simulink model "SH_control_harness1"  (R2023b)
settings: Solver=VariableStepAuto  StartTime=0.0  StopTime=inf  RelTol=1e-3
settings Model: Creator=Veimar  LastModifiedBy=Veimar

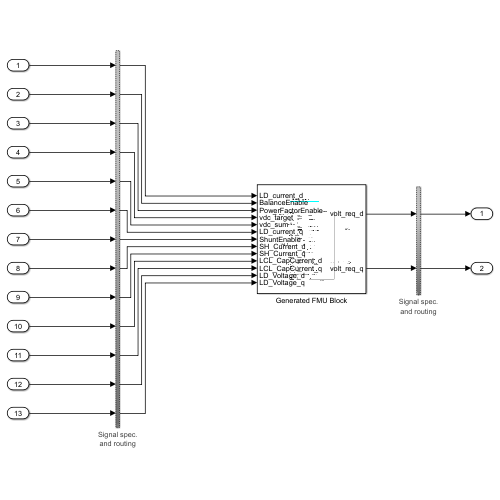
[thumbnail: Simulink's stored preview of the top-level diagram]
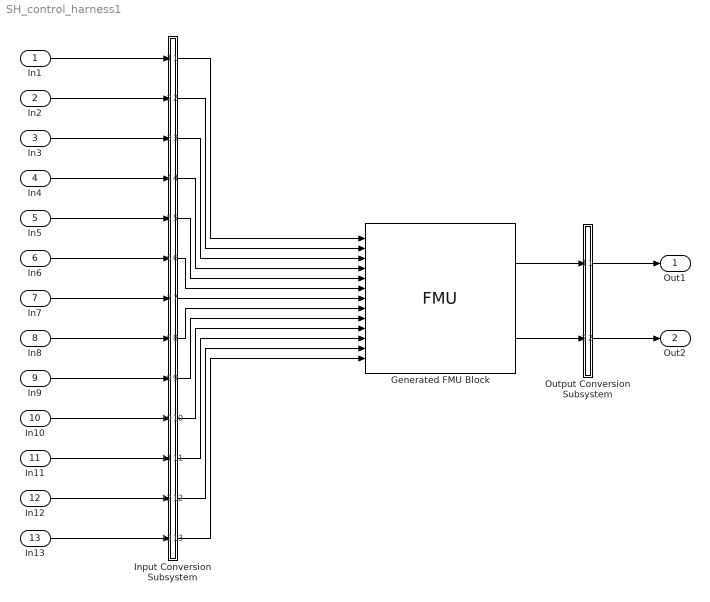
== system SH_control_harness1 ==
  In1 : Inport  OutDataTypeStr=double  PortDimensions=[3]  SampleTime=0.00026667
  In2 : Inport  Port=2  OutDataTypeStr=int32  PortDimensions=[1]  SampleTime=0.00026667
  In3 : Inport  Port=3  OutDataTypeStr=int32  PortDimensions=[1]  SampleTime=0.00026667
  In4 : Inport  Port=4  OutDataTypeStr=double  PortDimensions=[1]  SampleTime=0.00026667
  In5 : Inport  Port=5  OutDataTypeStr=double  PortDimensions=[1]  SampleTime=0.00026667
  In6 : Inport  Port=6  OutDataTypeStr=double  PortDimensions=[3]  SampleTime=0.00026667
  In7 : Inport  Port=7  OutDataTypeStr=int32  PortDimensions=[1]  SampleTime=0.00026667
  In8 : Inport  Port=8  OutDataTypeStr=double  PortDimensions=[3]  SampleTime=0.00026667
  In9 : Inport  Port=9  OutDataTypeStr=double  PortDimensions=[3]  SampleTime=0.00026667
  In10 : Inport  Port=10  OutDataTypeStr=double  PortDimensions=[3]  SampleTime=0.00026667
  In11 : Inport  Port=11  OutDataTypeStr=double  PortDimensions=[3]  SampleTime=0.00026667
  In12 : Inport  Port=12  OutDataTypeStr=double  PortDimensions=[3]  SampleTime=0.00026667
  In13 : Inport  Port=13  OutDataTypeStr=double  PortDimensions=[3]  SampleTime=0.00026667
  Generated FMU Block : FMU  FMUName=SH_control  FMUMode=CoSimulation  FMUSampleTime=0.00026667  FMUCreateBusObject=off  FMUInitializeEnumObject=off
      mask Type: SH_control [Co-Simulation, v2.0]
      mask Display:
      | if (exist([Simulink.fileGenControl('get','CacheFolder') '\slprj\_fmu\569492d8a8441ae19fe950d3b8ff40c2\SH_control\model.png'],'file'))
      |     image([Simulink.fileGenControl('get','CacheFolder') '\slprj\_fmu\569492d8a8441ae19fe950d3b8ff40c2\SH_control\model.png']);
      | else
      |     disp('SH_control');
      | end
      | port_label('output',1,'volt_req_d');
      | port_label('output',2,'volt_req_q');
      | port_label('input',1,'LD_current_d');
      | port_label('input',2,'BalanceEnable');
      | port_label('input',3,'PowerFactorEnable');
      | port_label('input',4,'vdc_target');
      | port_label('input',5,'vdc_sum');
      | port_label('input',6,'LD_current_q');
      | port_label('input',7,'ShuntEnable');
      | port_label('input',8,'SH_Current_d');
      | port_label('input',9,'SH_Current_q');
      | port_label('input',10,'LCL_CapCurrent_d');
      | port_label('input',11,'LCL_CapCurrent_q');
      | port_label('input',12,'LD_Voltage_d');
      | port_label('input',13,'LD_Voltage_q');
  Input Conversion Subsystem : Subsystem  Tag=__SLT_ICS__  Description=|
      | Signal spec.
      | and routing
      settings: AttributesFormatString=%<Description>
  Output Conversion Subsystem : Subsystem  Tag=__SLT_OCS__  Description=|
      | Signal spec.
      | and routing
      settings: AttributesFormatString=%<Description>
  Out1 : Outport
  Out2 : Outport  Port=2
  wires:
  In1/1 -> Input Conversion Subsystem/1(Inport_1)
  In2/1 -> Input Conversion Subsystem/2(Inport_2)
  In3/1 -> Input Conversion Subsystem/3(Inport_3)
  In4/1 -> Input Conversion Subsystem/4(Inport_4)
  In5/1 -> Input Conversion Subsystem/5(Inport_5)
  In6/1 -> Input Conversion Subsystem/6(Inport_6)
  In7/1 -> Input Conversion Subsystem/7(Inport_7)
  In8/1 -> Input Conversion Subsystem/8(Inport_8)
  In9/1 -> Input Conversion Subsystem/9(Inport_9)
  In10/1 -> Input Conversion Subsystem/10(Inport_10)
  In11/1 -> Input Conversion Subsystem/11(Inport_11)
  In12/1 -> Input Conversion Subsystem/12(Inport_12)
  In13/1 -> Input Conversion Subsystem/13(Inport_13)
  Output Conversion Subsystem/1(Outport_1) -> Out1/1
  Output Conversion Subsystem/2(Outport_2) -> Out2/1
  Input Conversion Subsystem/1(Outport_1) -> Generated FMU Block/1
  Input Conversion Subsystem/2(Outport_2) -> Generated FMU Block/2
  Input Conversion Subsystem/3(Outport_3) -> Generated FMU Block/3
  Input Conversion Subsystem/4(Outport_4) -> Generated FMU Block/4
  Input Conversion Subsystem/5(Outport_5) -> Generated FMU Block/5
  Input Conversion Subsystem/6(Outport_6) -> Generated FMU Block/6
  Input Conversion Subsystem/7(Outport_7) -> Generated FMU Block/7
  Input Conversion Subsystem/8(Outport_8) -> Generated FMU Block/8
  Input Conversion Subsystem/9(Outport_9) -> Generated FMU Block/9
  Input Conversion Subsystem/10(Outport_10) -> Generated FMU Block/10
  Input Conversion Subsystem/11(Outport_11) -> Generated FMU Block/11
  Input Conversion Subsystem/12(Outport_12) -> Generated FMU Block/12
  Input Conversion Subsystem/13(Outport_13) -> Generated FMU Block/13
  Generated FMU Block/1 -> Output Conversion Subsystem/1(Inport_1)
  Generated FMU Block/2 -> Output Conversion Subsystem/2(Inport_2)

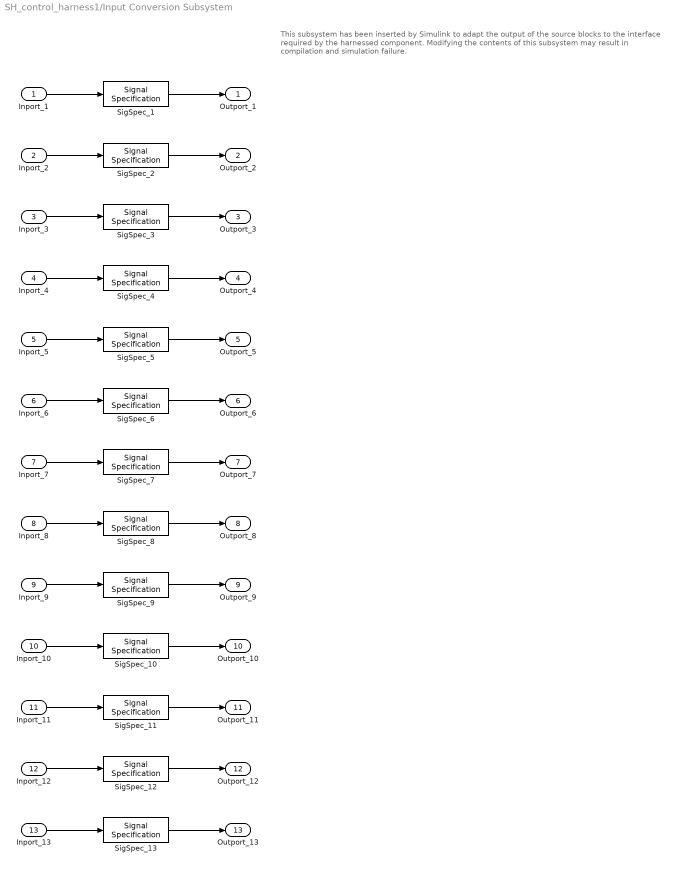
== system SH_control_harness1/Input Conversion Subsystem ==
  note: This subsystem has been inserted by Simulink to adapt the output of the source blocks to the interface required by the harnessed component.
      |  Modifying the contents of this subsystem may result in compilation and simulation failure.
  Inport_1 : Inport
  Inport_2 : Inport  Port=2
  Inport_3 : Inport  Port=3
  Inport_4 : Inport  Port=4
  Inport_5 : Inport  Port=5
  Inport_6 : Inport  Port=6
  Inport_7 : Inport  Port=7
  Inport_8 : Inport  Port=8
  Inport_9 : Inport  Port=9
  Inport_10 : Inport  Port=10
  Inport_11 : Inport  Port=11
  Inport_12 : Inport  Port=12
  Inport_13 : Inport  Port=13
  SigSpec_{1,6,8..13} (8 alike) : SignalSpecification  OutDataTypeStr=double  Dimensions=[3]  SampleTime=0.00026667
  SigSpec_2 : SignalSpecification  OutDataTypeStr=int32  Dimensions=[1]  SampleTime=0.00026667
  SigSpec_3 : SignalSpecification  OutDataTypeStr=int32  Dimensions=[1]  SampleTime=0.00026667
  SigSpec_4 : SignalSpecification  OutDataTypeStr=double  Dimensions=[1]  SampleTime=0.00026667
  SigSpec_5 : SignalSpecification  OutDataTypeStr=double  Dimensions=[1]  SampleTime=0.00026667
  SigSpec_7 : SignalSpecification  OutDataTypeStr=int32  Dimensions=[1]  SampleTime=0.00026667
  Outport_1 : Outport
  Outport_2 : Outport  Port=2
  Outport_3 : Outport  Port=3
  Outport_4 : Outport  Port=4
  Outport_5 : Outport  Port=5
  Outport_6 : Outport  Port=6
  Outport_7 : Outport  Port=7
  Outport_8 : Outport  Port=8
  Outport_9 : Outport  Port=9
  Outport_10 : Outport  Port=10
  Outport_11 : Outport  Port=11
  Outport_12 : Outport  Port=12
  Outport_13 : Outport  Port=13
  wires:
  SigSpec_1/1 -> Outport_1/1
  Inport_1/1 -> SigSpec_1/1
  SigSpec_2/1 -> Outport_2/1
  Inport_2/1 -> SigSpec_2/1
  SigSpec_3/1 -> Outport_3/1
  Inport_3/1 -> SigSpec_3/1
  SigSpec_4/1 -> Outport_4/1
  Inport_4/1 -> SigSpec_4/1
  SigSpec_5/1 -> Outport_5/1
  Inport_5/1 -> SigSpec_5/1
  SigSpec_6/1 -> Outport_6/1
  Inport_6/1 -> SigSpec_6/1
  SigSpec_7/1 -> Outport_7/1
  Inport_7/1 -> SigSpec_7/1
  SigSpec_8/1 -> Outport_8/1
  Inport_8/1 -> SigSpec_8/1
  SigSpec_9/1 -> Outport_9/1
  Inport_9/1 -> SigSpec_9/1
  SigSpec_10/1 -> Outport_10/1
  Inport_10/1 -> SigSpec_10/1
  SigSpec_11/1 -> Outport_11/1
  Inport_11/1 -> SigSpec_11/1
  SigSpec_12/1 -> Outport_12/1
  Inport_12/1 -> SigSpec_12/1
  SigSpec_13/1 -> Outport_13/1
  Inport_13/1 -> SigSpec_13/1

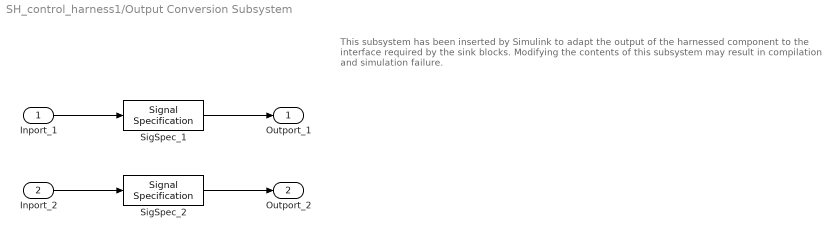
== system SH_control_harness1/Output Conversion Subsystem ==
  note: This subsystem has been inserted by Simulink to adapt the output of the harnessed component to the interface required by the sink blocks.
      |  Modifying the contents of this subsystem may result in compilation and simulation failure.
  Inport_1 : Inport
  Inport_2 : Inport  Port=2
  SigSpec_1 : SignalSpecification  OutDataTypeStr=double  Dimensions=[3]  SampleTime=0.00026667
  SigSpec_2 : SignalSpecification  OutDataTypeStr=double  Dimensions=[3]  SampleTime=0.00026667
  Outport_1 : Outport
  Outport_2 : Outport  Port=2
  wires:
  Inport_1/1 -> SigSpec_1/1
  SigSpec_1/1 -> Outport_1/1
  Inport_2/1 -> SigSpec_2/1
  SigSpec_2/1 -> Outport_2/1
